simulink model "SimulationForFigure7"  (R2024a)
settings: Solver=ode23tb  StartTime=0.0  StopTime=10.0  RelTol=1e-3
values from neighbouring files (symbols this model uses):
  C_f = 4e-3    (= 0.004)    [necessary_parameter_for_GFM.m]
  C_f_base = 1/(w_nom*Z_base)    (= 0.039788735773)    [necessary_parameter_for_GFM.m]
  kpw = (0.5*2*pi)/1e6    (= 3.14159265359e-06)    [necessary_parameter_for_GFM.m]
  kqv = 20/(1e6)    (= 2e-05)    [necessary_parameter_for_GFM.m]
  L_f = 8e-6    (= 8e-06)    [necessary_parameter_for_GFM.m]
  L_f_base = Z_base/w_nom    (= 0.000254647908947)    [necessary_parameter_for_GFM.m]
  L_g = Length*L_g_per_km    (= 0.005)    [necessary_parameter_for_GFM.m]
  R_f = 1e-4    (= 0.0001)    [necessary_parameter_for_GFM.m]
  R_g = Length*R_g_per_km    (= 0.75)    [necessary_parameter_for_GFM.m]
  V_dc = 1000    [necessary_parameter_for_GFM.m]
  w_nom = 2*pi*f_nom    (= 314.159265359)    [necessary_parameter_for_GFM.m]
libraries: spsabctodq0Lib x8, slpidlib x8, dspstat3 x8, spsThreePhaseSeriesRLCLoadLib x8, spsVoltageMeasurementLib x8, spsThreePhaseSeriesRLCBranchLib x6, spsThreePhaseBreakerLib x6, spsPower3phInstantaneousLib x4, spsThreePhaseVIMeasurementLib x4, cstblocks x4, spsDCVoltageSourceLib x2, spsdq0toabcLib x2
(part 1 of 2)
settings Model: Creator=USER  LastModifiedBy=USER
settings DebuggingCC: AlgebraicLoopMsg=none

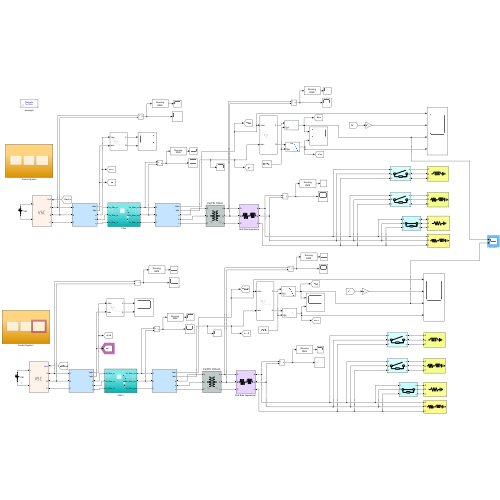
[thumbnail: Simulink's stored preview of the top-level diagram]
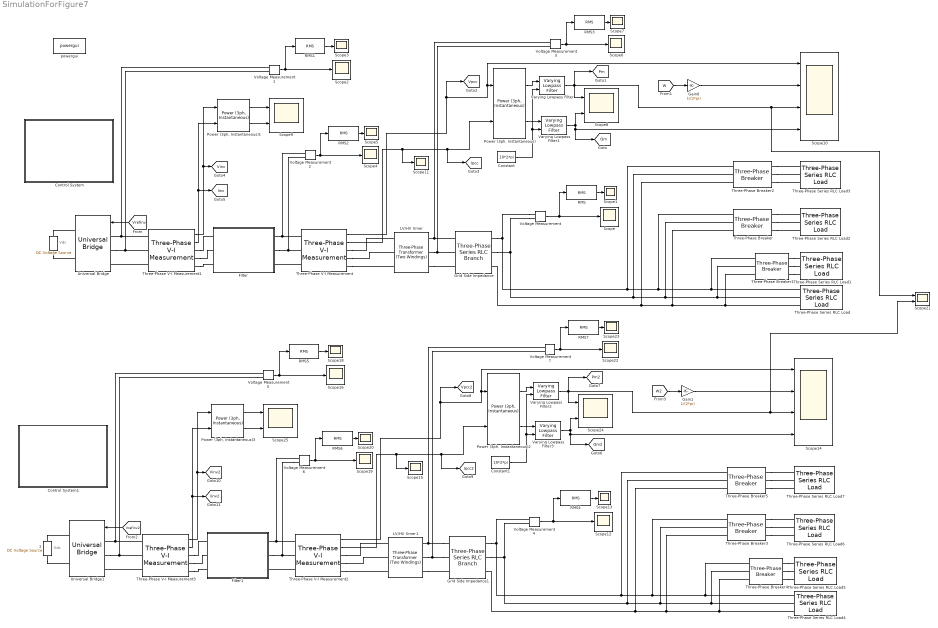
== system SimulationForFigure7 ==
  note: Vdc
  note: Vdc
  "               " : spsDCVoltageSourceLib/DC Voltage Source  Amplitude=V_dc  Measurements=None
  "               1" : spsDCVoltageSourceLib/DC Voltage Source  Amplitude=V_dc  Measurements=None
  Constant : Constant  Value=10*2*pi
  Constant1 : Constant  Value=10*2*pi
  Control System : Subsystem
  Control System1 : Subsystem
  Filter : Subsystem
  Filter1 : Subsystem
  Gain1 : Gain  Gain=1/(2*pi)
  Gain6 : Gain  Gain=1/(2*pi)
  Grid Side Impedance : spsThreePhaseSeriesRLCBranchLib/Three-Phase Series RLC Branch  LConnTagsString=A|B|C  RConnTagsString=A|B|C  BranchType=RL  Resistance=R_g  Inductance=L_g  Capacitance=1e-6  Measurements=None
  Grid Side Impedance1 : spsThreePhaseSeriesRLCBranchLib/Three-Phase Series RLC Branch  LConnTagsString=A|B|C  RConnTagsString=A|B|C  BranchType=RL  Resistance=R_g  Inductance=L_g  Capacitance=1e-6  Measurements=None
  LV/HV Xmer : spsThreePhaseTransformerTwoWindingsLib/Three-Phase Transformer (Two Windings)  Winding1Connection=Yg  Winding2Connection=Yg  CoreType=Three single-phase transformers  SetSaturation=off  Hysteresis=off  DataFile='hysteresis'  SetInitialFlux=off  Measurements=None  UNITS=SI  NominalPower=[ 2000000 50 ]  Winding1=[400 0 0]  Winding2=[33000 0 0]  Rm=inf  Lm=inf  L0=0.5  Saturation=[0 0;20.412 1.2475;4082.5 1.4554]  InitialFluxes=[ 0.8 , -0.8 , 0.7 ]  BreakLoop=off  DiscreteSolver=Trapezoidal iterative  DataType=on  TransfoNumber=0
  LV/HV Xmer1 : spsThreePhaseTransformerTwoWindingsLib/Three-Phase Transformer (Two Windings)  Winding1Connection=Yg  Winding2Connection=Yg  CoreType=Three single-phase transformers  SetSaturation=off  Hysteresis=off  DataFile='hysteresis'  SetInitialFlux=off  Measurements=None  UNITS=SI  NominalPower=[ 2000000 50 ]  Winding1=[400 0 0]  Winding2=[33000 0 0]  Rm=inf  Lm=inf  L0=0.5  Saturation=[0 0;20.412 1.2475;4082.5 1.4554]  InitialFluxes=[ 0.8 , -0.8 , 0.7 ]  BreakLoop=off  DiscreteSolver=Trapezoidal iterative  DataType=on  TransfoNumber=0
  Power (3ph, Instantaneous){,1..3} (4 alike) : spsPower3phInstantaneousLib/Power (3ph, Instantaneous)
  RMS{,1..7} (8 alike) : dspstat3/RMS  run=on  directionMode=Each column  dimension=1  InputProcessing=Columns as channels (frame based)  reset_popup=None
  Scope{,1..7,11..13,15..16,18..20,22..23} (18 alike) : Scope
  Scope10 : Scope  NumInputPorts=4
  Scope14 : Scope  NumInputPorts=4
  Scope{8..9,21,24..25} (5 alike) : Scope  NumInputPorts=2
  Three-Phase Series RLC Load : spsThreePhaseSeriesRLCLoadLib/Three-Phase Series RLC Load  LConnTagsString=A|B|C  Configuration=Y (grounded)  NominalVoltage=33000  Vabc=[1e3 1e3 1e3]  Vabcp=[1e3 1e3 1e3]  NominalFrequency=50  UnbalancedPower=off  ActivePower=0.9e6  InductivePower=4e5  CapacitivePower=0  Pabc=[10e3 9e3 11e3]  QLabc=[100 90 110]  QCabc=[100 90 110]  Pabcp=[10e3 9e3 11e3]  QLabcp=[100 90 110]  QCabcp=[100 90 110]  Measurements=None  LoadType=constant Z
  Three-Phase Series RLC Load1 : spsThreePhaseSeriesRLCLoadLib/Three-Phase Series RLC Load  LConnTagsString=A|B|C  Configuration=Y (grounded)  NominalVoltage=33000  Vabc=[1e3 1e3 1e3]  Vabcp=[1e3 1e3 1e3]  NominalFrequency=50  UnbalancedPower=off  ActivePower=0.1e6  InductivePower=0  CapacitivePower=0  Pabc=[10e3 9e3 11e3]  QLabc=[100 90 110]  QCabc=[100 90 110]  Pabcp=[10e3 9e3 11e3]  QLabcp=[100 90 110]  QCabcp=[100 90 110]  Measurements=None  LoadType=constant Z
  Three-Phase Series RLC Load2 : spsThreePhaseSeriesRLCLoadLib/Three-Phase Series RLC Load  LConnTagsString=A|B|C  Configuration=Y (grounded)  NominalVoltage=33000  Vabc=[1e3 1e3 1e3]  Vabcp=[1e3 1e3 1e3]  NominalFrequency=50  UnbalancedPower=off  ActivePower=0.2e6  InductivePower=4e5  CapacitivePower=0  Pabc=[10e3 9e3 11e3]  QLabc=[100 90 110]  QCabc=[100 90 110]  Pabcp=[10e3 9e3 11e3]  QLabcp=[100 90 110]  QCabcp=[100 90 110]  Measurements=None  LoadType=constant Z
  Three-Phase Series RLC Load3 : spsThreePhaseSeriesRLCLoadLib/Three-Phase Series RLC Load  LConnTagsString=A|B|C  Configuration=Y (grounded)  NominalVoltage=33000  Vabc=[1e3 1e3 1e3]  Vabcp=[1e3 1e3 1e3]  NominalFrequency=50  UnbalancedPower=off  ActivePower=0  InductivePower=1e5  CapacitivePower=0  Pabc=[10e3 9e3 11e3]  QLabc=[100 90 110]  QCabc=[100 90 110]  Pabcp=[10e3 9e3 11e3]  QLabcp=[100 90 110]  QCabcp=[100 90 110]  Measurements=None  LoadType=constant Z
  Three-Phase Series RLC Load4 : spsThreePhaseSeriesRLCLoadLib/Three-Phase Series RLC Load  LConnTagsString=A|B|C  Configuration=Y (grounded)  NominalVoltage=33000  Vabc=[1e3 1e3 1e3]  Vabcp=[1e3 1e3 1e3]  NominalFrequency=50  UnbalancedPower=off  ActivePower=0.9e6  InductivePower=4e5  CapacitivePower=0  Pabc=[10e3 9e3 11e3]  QLabc=[100 90 110]  QCabc=[100 90 110]  Pabcp=[10e3 9e3 11e3]  QLabcp=[100 90 110]  QCabcp=[100 90 110]  Measurements=None  LoadType=constant Z
  Three-Phase Series RLC Load5 : spsThreePhaseSeriesRLCLoadLib/Three-Phase Series RLC Load  LConnTagsString=A|B|C  Configuration=Y (grounded)  NominalVoltage=33000  Vabc=[1e3 1e3 1e3]  Vabcp=[1e3 1e3 1e3]  NominalFrequency=50  UnbalancedPower=off  ActivePower=0.1e6  InductivePower=0  CapacitivePower=0  Pabc=[10e3 9e3 11e3]  QLabc=[100 90 110]  QCabc=[100 90 110]  Pabcp=[10e3 9e3 11e3]  QLabcp=[100 90 110]  QCabcp=[100 90 110]  Measurements=None  LoadType=constant Z
  Three-Phase Series RLC Load6 : spsThreePhaseSeriesRLCLoadLib/Three-Phase Series RLC Load  LConnTagsString=A|B|C  Configuration=Y (grounded)  NominalVoltage=33000  Vabc=[1e3 1e3 1e3]  Vabcp=[1e3 1e3 1e3]  NominalFrequency=50  UnbalancedPower=off  ActivePower=0.2e6  InductivePower=4e5  CapacitivePower=0  Pabc=[10e3 9e3 11e3]  QLabc=[100 90 110]  QCabc=[100 90 110]  Pabcp=[10e3 9e3 11e3]  QLabcp=[100 90 110]  QCabcp=[100 90 110]  Measurements=None  LoadType=constant Z
  Three-Phase Series RLC Load7 : spsThreePhaseSeriesRLCLoadLib/Three-Phase Series RLC Load  LConnTagsString=A|B|C  Configuration=Y (grounded)  NominalVoltage=33000  Vabc=[1e3 1e3 1e3]  Vabcp=[1e3 1e3 1e3]  NominalFrequency=50  UnbalancedPower=off  ActivePower=0  InductivePower=1e5  CapacitivePower=0  Pabc=[10e3 9e3 11e3]  QLabc=[100 90 110]  QCabc=[100 90 110]  Pabcp=[10e3 9e3 11e3]  QLabcp=[100 90 110]  QCabcp=[100 90 110]  Measurements=None  LoadType=constant Z
  Three-Phase V-I Measurement{,1..3} (4 alike) : spsThreePhaseVIMeasurementLib/Three-Phase V-I Measurement  VoltageMeasurement=phase-to-ground  SetLabelV=off  LabelV=Vabc  Vpu=off  VpuLL=off  CurrentMeasurement=yes  SetLabelI=off  LabelI=Iabc  Ipu=off  Pbase=100e6  Vbase=500e3  OutputType=Complex  PhasorSimulation=off  PSBequivalent=0
  Three-Phase Breaker : spsThreePhaseBreakerLib/Three-Phase Breaker  InitialState=open  SwitchA=on  SwitchB=on  SwitchC=on  SwitchTimes="[2  3]"  External=off  BreakerResistance=0.001  SnubberResistance=1e6  SnubberCapacitance=inf  Measurements=None
  Three-Phase Breaker1 : spsThreePhaseBreakerLib/Three-Phase Breaker  InitialState=closed  SwitchA=on  SwitchB=on  SwitchC=on  SwitchTimes=[6 8]  External=off  BreakerResistance=0.001  SnubberResistance=1e6  SnubberCapacitance=inf  Measurements=None
  Three-Phase Breaker2 : spsThreePhaseBreakerLib/Three-Phase Breaker  InitialState=open  SwitchA=on  SwitchB=on  SwitchC=on  SwitchTimes="[4  5]"  External=off  BreakerResistance=0.001  SnubberResistance=1e6  SnubberCapacitance=inf  Measurements=None
  Three-Phase Breaker3 : spsThreePhaseBreakerLib/Three-Phase Breaker  InitialState=open  SwitchA=on  SwitchB=on  SwitchC=on  SwitchTimes="[2  3]"  External=off  BreakerResistance=0.001  SnubberResistance=1e6  SnubberCapacitance=inf  Measurements=None
  Three-Phase Breaker4 : spsThreePhaseBreakerLib/Three-Phase Breaker  InitialState=closed  SwitchA=on  SwitchB=on  SwitchC=on  SwitchTimes=[6 8]  External=off  BreakerResistance=0.001  SnubberResistance=1e6  SnubberCapacitance=inf  Measurements=None
  Three-Phase Breaker5 : spsThreePhaseBreakerLib/Three-Phase Breaker  InitialState=open  SwitchA=on  SwitchB=on  SwitchC=on  SwitchTimes="[4  5]"  External=off  BreakerResistance=0.001  SnubberResistance=1e6  SnubberCapacitance=inf  Measurements=None
  Universal Bridge : spsUniversalBridgeLib/Universal Bridge  Arms=3  SnubberResistance=1e5  SnubberCapacitance=inf  Device=Average-model based VSC  Ron=1e-3  Lon=0  ForwardVoltages="[  0  0  ]"  ForwardVoltage=0  GTOparameters=[ 10e-6 , 20e-6 ]  IGBTparameters=[ 1e-6 , 2e-6 ]  Measurements=None  Measurements_2=None  converterType=Rectifier
  Universal Bridge1 : spsUniversalBridgeLib/Universal Bridge  Arms=3  SnubberResistance=1e5  SnubberCapacitance=inf  Device=Average-model based VSC  Ron=1e-3  Lon=0  ForwardVoltages="[  0  0  ]"  ForwardVoltage=0  GTOparameters=[ 10e-6 , 20e-6 ]  IGBTparameters=[ 1e-6 , 2e-6 ]  Measurements=None  Measurements_2=None  converterType=Rectifier
  Varying Lowpass Filter{,1..3} (4 alike) : cstblocks/Linear Parameter Varying/Varying Lowpass Filter  N=2
  Voltage Measurement{,1..7} (8 alike) : spsVoltageMeasurementLib/Voltage Measurement  PhasorSimulation=off  OutputType=Complex  PSBequivalent=0
  powergui : sps_lib/powergui  Priority=1  SimulationMode=Discrete  SampleTime=1e-5  frequency=60  Iterations=50  frequencyindice=0  Pbase=100e6  ErrMax=1e-4  UnitsV=kV  UnitsW=MW  buscounter=0  FunctionMessages=off  echomessages=off  EnableUseOfTLC=off  CurrentSourceSwitches=off  DisableSnubberDevices=off  DisableRonSwitches=off  DisableVfSwitches=off  DisplayEquations=off  AutomaticDiscreteSolvers=off  SolverType=Tustin/Backward Euler (TBE)  Interpol=off  ExternalGateDelay=off  methode=off  Ts=100  x0status=blocks  SPID=on  SwTol=0  HookPort=off  NonlinearTolerance=1e-4  nMaxIteration=100  ContinueOnMaxIteration=off  RestoreLinks=warning  ResistiveCurrentMeasurement=off  Frange=[0:2:500]  Ylog=off  Xlog=on  ShowGrid=off  save=off  variable=ZData  structure=0  ZoomFFT=off  StartTime=0.0  cycles=1  DisplayStyle=1  fundamental=60  FreqAxis=off  MaxFrequency=1000  frequencyindicesteady=1  RmsSteady=1  display=off
  tag scope: Iinv2=global, Iinv=global, Ipcc2=global, Ipcc=global, Pm2=global, Pm=global, Qm2=global, Qm=global, Vinv2=global, Vinv=global, Vpcc2=global, Vpcc=global
  wires:
  Voltage Measurement1/1 -> RMS1/1, Scope2/1
  RMS/1 -> Scope1/1
  Voltage Measurement/1 -> RMS/1, Scope/1
  RMS2/1 -> Scope5/1
  [Vrefinv] -> Universal Bridge/1
  RMS1/1 -> Scope3/1
  RMS3/1 -> Scope7/1
  Voltage Measurement3/1 -> RMS3/1, Scope6/1
  Voltage Measurement2/1 -> RMS2/1, Scope4/1
  [W] -> Gain6/1
  Three-Phase V-I Measurement/1 -> [Vpcc], Scope10/1, "Power (3ph, Instantaneous)"/1
  Three-Phase V-I Measurement/2 -> Scope11/1, [Ipcc], "Power (3ph, Instantaneous)"/2
  Three-Phase V-I Measurement1/1 -> "Power (3ph, Instantaneous)1"/1, [Vinv]
  Three-Phase V-I Measurement1/2 -> "Power (3ph, Instantaneous)1"/2, [Iinv]
  "Power (3ph, Instantaneous)1"/1 -> Scope9/1
  "Power (3ph, Instantaneous)1"/2 -> Scope9/2
  Gain6/1 -> Scope10/2
  "Power (3ph, Instantaneous)"/2 -> Varying Lowpass Filter1/1
  Varying Lowpass Filter1/1 -> Scope10/4, [Qm], Scope8/2
  Varying Lowpass Filter/1 -> Scope10/3, Scope21/1, Scope8/1, [Pm]
  "Power (3ph, Instantaneous)"/1 -> Varying Lowpass Filter/1
  Constant/1 -> Varying Lowpass Filter1/2, Varying Lowpass Filter/2
  "Power (3ph, Instantaneous)2"/1 -> Varying Lowpass Filter2/1
  Varying Lowpass Filter2/1 -> Scope21/2, Scope14/3, Scope24/1, [Pm2]
  Three-Phase V-I Measurement3/2 -> "Power (3ph, Instantaneous)3"/2, [Iinv2]
  Three-Phase V-I Measurement2/2 -> Scope15/1, [Ipcc2], "Power (3ph, Instantaneous)2"/2
  Three-Phase V-I Measurement2/1 -> [Vpcc2], Scope14/1, "Power (3ph, Instantaneous)2"/1
  RMS4/1 -> Scope13/1
  RMS7/1 -> Scope23/1
  Voltage Measurement4/1 -> RMS4/1, Scope12/1
  Voltage Measurement5/1 -> RMS5/1, Scope16/1
  RMS6/1 -> Scope20/1
  RMS5/1 -> Scope18/1
  Gain1/1 -> Scope14/2
  Constant1/1 -> Varying Lowpass Filter3/2, Varying Lowpass Filter2/2
  Voltage Measurement6/1 -> RMS6/1, Scope19/1
  Varying Lowpass Filter3/1 -> Scope14/4, [Qm2], Scope24/2
  [W2] -> Gain1/1
  Three-Phase V-I Measurement3/1 -> "Power (3ph, Instantaneous)3"/1, [Vinv2]
  Voltage Measurement7/1 -> RMS7/1, Scope22/1
  "Power (3ph, Instantaneous)3"/2 -> Scope25/2
  "Power (3ph, Instantaneous)2"/2 -> Varying Lowpass Filter3/1
  "Power (3ph, Instantaneous)3"/1 -> Scope25/1
  [Vrefinv2] -> Universal Bridge1/1
  connections:
  Voltage Measurement/LConn2 -- Three-Phase Breaker2/LConn2 -- Three-Phase Breaker/LConn2 -- Three-Phase Series RLC Load/LConn2 -- Three-Phase Breaker1/LConn2 -- Grid Side Impedance/RConn2
  Voltage Measurement1/LConn1 -- Universal Bridge/LConn1 -- Three-Phase V-I Measurement1/LConn1
  Universal Bridge/LConn2 -- Three-Phase V-I Measurement1/LConn2 -- Voltage Measurement1/LConn2
  Voltage Measurement/LConn1 -- Three-Phase Breaker2/LConn1 -- Three-Phase Series RLC Load/LConn1 -- Three-Phase Breaker1/LConn1 -- Three-Phase Breaker/LConn1 -- Grid Side Impedance/RConn1
  Filter/RConn2 -- Three-Phase V-I Measurement/LConn2 -- Voltage Measurement2/LConn2
  Voltage Measurement2/LConn1 -- Three-Phase V-I Measurement/LConn1 -- Filter/RConn1
  "               "/LConn1 -- Universal Bridge/RConn2
  Three-Phase V-I Measurement/LConn3 -- Filter/RConn3
  "               "/RConn1 -- Universal Bridge/RConn1
  Three-Phase V-I Measurement/RConn1 -- LV/HV Xmer/LConn1
  Three-Phase V-I Measurement/RConn2 -- LV/HV Xmer/LConn2
  Three-Phase V-I Measurement/RConn3 -- LV/HV Xmer/LConn3
  LV/HV Xmer/RConn1 -- Voltage Measurement3/LConn1 -- Grid Side Impedance/LConn1
  LV/HV Xmer/RConn2 -- Voltage Measurement3/LConn2 -- Grid Side Impedance/LConn2
  LV/HV Xmer/RConn3 -- Grid Side Impedance/LConn3
  Three-Phase V-I Measurement1/LConn3 -- Universal Bridge/LConn3
  Three-Phase V-I Measurement1/RConn1 -- Filter/LConn1
  Three-Phase V-I Measurement1/RConn2 -- Filter/LConn2
  Three-Phase V-I Measurement1/RConn3 -- Filter/LConn3
  Three-Phase Breaker/LConn3 -- Three-Phase Series RLC Load/LConn3 -- Three-Phase Breaker1/LConn3 -- Three-Phase Breaker2/LConn3 -- Grid Side Impedance/RConn3
  Three-Phase Breaker/RConn3 -- Three-Phase Series RLC Load2/LConn3
  Three-Phase Breaker1/RConn1 -- Three-Phase Series RLC Load1/LConn1
  Three-Phase Breaker1/RConn2 -- Three-Phase Series RLC Load1/LConn2
  Three-Phase Breaker/RConn2 -- Three-Phase Series RLC Load2/LConn2
  Three-Phase Breaker1/RConn3 -- Three-Phase Series RLC Load1/LConn3
  Three-Phase Breaker/RConn1 -- Three-Phase Series RLC Load2/LConn1
  Three-Phase Breaker2/RConn1 -- Three-Phase Series RLC Load3/LConn1
  Three-Phase Breaker2/RConn2 -- Three-Phase Series RLC Load3/LConn2
  Three-Phase Breaker2/RConn3 -- Three-Phase Series RLC Load3/LConn3
  Filter1/RConn1 -- Voltage Measurement6/LConn1 -- Three-Phase V-I Measurement2/LConn1
  Three-Phase Breaker3/LConn1 -- Voltage Measurement4/LConn1 -- Grid Side Impedance1/RConn1 -- Three-Phase Breaker5/LConn1 -- Three-Phase Series RLC Load4/LConn1 -- Three-Phase Breaker4/LConn1
  Voltage Measurement5/LConn2 -- Universal Bridge1/LConn2 -- Three-Phase V-I Measurement3/LConn2
  Grid Side Impedance1/RConn2 -- Voltage Measurement4/LConn2 -- Three-Phase Breaker5/LConn2 -- Three-Phase Breaker3/LConn2 -- Three-Phase Series RLC Load4/LConn2 -- Three-Phase Breaker4/LConn2
  Grid Side Impedance1/LConn2 -- LV/HV Xmer1/RConn2 -- Voltage Measurement7/LConn2
  Grid Side Impedance1/LConn1 -- LV/HV Xmer1/RConn1 -- Voltage Measurement7/LConn1
  Three-Phase V-I Measurement3/LConn1 -- Voltage Measurement5/LConn1 -- Universal Bridge1/LConn1
  Three-Phase Breaker4/LConn3 -- Three-Phase Series RLC Load4/LConn3 -- Three-Phase Breaker5/LConn3 -- Grid Side Impedance1/RConn3 -- Three-Phase Breaker3/LConn3
  Voltage Measurement6/LConn2 -- Filter1/RConn2 -- Three-Phase V-I Measurement2/LConn2
  Three-Phase V-I Measurement3/RConn1 -- Filter1/LConn1
  Three-Phase V-I Measurement3/RConn3 -- Filter1/LConn3
  Three-Phase Breaker5/RConn3 -- Three-Phase Series RLC Load7/LConn3
  "               1"/LConn1 -- Universal Bridge1/RConn2
  "               1"/RConn1 -- Universal Bridge1/RConn1
  Three-Phase V-I Measurement2/RConn1 -- LV/HV Xmer1/LConn1
  LV/HV Xmer1/RConn3 -- Grid Side Impedance1/LConn3
  Three-Phase Breaker3/RConn2 -- Three-Phase Series RLC Load6/LConn2
  Three-Phase Breaker5/RConn1 -- Three-Phase Series RLC Load7/LConn1
  Three-Phase Breaker4/RConn3 -- Three-Phase Series RLC Load5/LConn3
  Three-Phase V-I Measurement3/LConn3 -- Universal Bridge1/LConn3
  Three-Phase Breaker4/RConn1 -- Three-Phase Series RLC Load5/LConn1
  Three-Phase Breaker5/RConn2 -- Three-Phase Series RLC Load7/LConn2
  Three-Phase Breaker4/RConn2 -- Three-Phase Series RLC Load5/LConn2
  Three-Phase V-I Measurement2/LConn3 -- Filter1/RConn3
  Three-Phase V-I Measurement3/RConn2 -- Filter1/LConn2
  Three-Phase V-I Measurement2/RConn2 -- LV/HV Xmer1/LConn2
  Three-Phase V-I Measurement2/RConn3 -- LV/HV Xmer1/LConn3
  Three-Phase Breaker3/RConn1 -- Three-Phase Series RLC Load6/LConn1
  Three-Phase Breaker3/RConn3 -- Three-Phase Series RLC Load6/LConn3

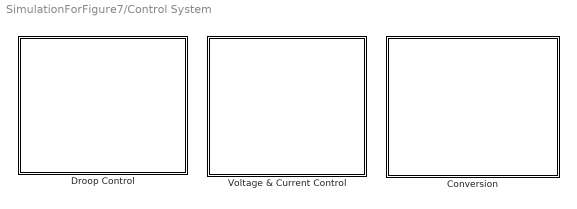
== system SimulationForFigure7/Control System ==
  Conversion : Subsystem
  Droop Control : Subsystem
  Voltage & Current Control : Subsystem

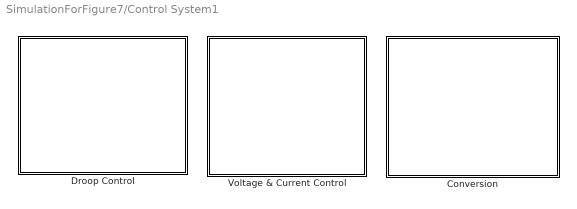
== system SimulationForFigure7/Control System1 ==
  Conversion : Subsystem
  Droop Control : Subsystem
  Voltage & Current Control : Subsystem

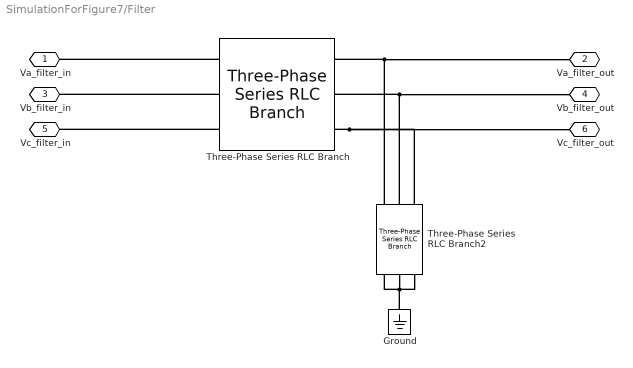
== system SimulationForFigure7/Filter ==
  Ground : spsGroundLib/Ground  LConnTagsString=a
  Three-Phase Series RLC Branch : spsThreePhaseSeriesRLCBranchLib/Three-Phase Series RLC Branch  LConnTagsString=A|B|C  RConnTagsString=A|B|C  BranchType=RL  Resistance=R_f  Inductance=L_f  Capacitance=1e-6  Measurements=None
  Three-Phase Series RLC Branch2 : spsThreePhaseSeriesRLCBranchLib/Three-Phase Series RLC Branch  LConnTagsString=A|B|C  RConnTagsString=A|B|C  BranchType=C  Resistance=1  Inductance=1e-3  Capacitance=C_f  Measurements=None
  Va_filter_in : PMIOPort  Side=Left
  Va_filter_out : PMIOPort  Port=2  Side=Right
  Vb_filter_in : PMIOPort  Port=3  Side=Left
  Vb_filter_out : PMIOPort  Port=4  Side=Right
  Vc_filter_in : PMIOPort  Port=5  Side=Left
  Vc_filter_out : PMIOPort  Port=6  Side=Right
  connections:
  Three-Phase Series RLC Branch2/RConn3 -- Ground/LConn1 -- Three-Phase Series RLC Branch2/RConn2 -- Three-Phase Series RLC Branch2/RConn1
  Three-Phase Series RLC Branch2/LConn2 -- Vb_filter_out/RConn1 -- Three-Phase Series RLC Branch/RConn2
  Three-Phase Series RLC Branch/RConn3 -- Vc_filter_out/RConn1 -- Three-Phase Series RLC Branch2/LConn3
  Three-Phase Series RLC Branch2/LConn1 -- Va_filter_out/RConn1 -- Three-Phase Series RLC Branch/RConn1
  Three-Phase Series RLC Branch/LConn3 -- Vc_filter_in/RConn1
  Three-Phase Series RLC Branch/LConn2 -- Vb_filter_in/RConn1
  Three-Phase Series RLC Branch/LConn1 -- Va_filter_in/RConn1

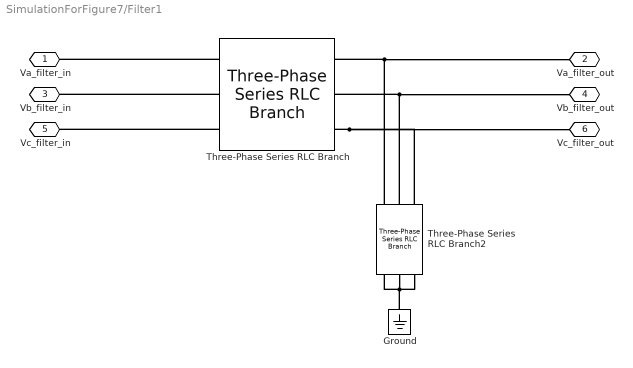
== system SimulationForFigure7/Filter1 ==
  Ground : spsGroundLib/Ground  LConnTagsString=a
  Three-Phase Series RLC Branch : spsThreePhaseSeriesRLCBranchLib/Three-Phase Series RLC Branch  LConnTagsString=A|B|C  RConnTagsString=A|B|C  BranchType=RL  Resistance=R_f  Inductance=L_f  Capacitance=1e-6  Measurements=None
  Three-Phase Series RLC Branch2 : spsThreePhaseSeriesRLCBranchLib/Three-Phase Series RLC Branch  LConnTagsString=A|B|C  RConnTagsString=A|B|C  BranchType=C  Resistance=1  Inductance=1e-3  Capacitance=C_f  Measurements=None
  Va_filter_in : PMIOPort  Side=Left
  Va_filter_out : PMIOPort  Port=2  Side=Right
  Vb_filter_in : PMIOPort  Port=3  Side=Left
  Vb_filter_out : PMIOPort  Port=4  Side=Right
  Vc_filter_in : PMIOPort  Port=5  Side=Left
  Vc_filter_out : PMIOPort  Port=6  Side=Right
  connections:
  Three-Phase Series RLC Branch2/RConn3 -- Ground/LConn1 -- Three-Phase Series RLC Branch2/RConn2 -- Three-Phase Series RLC Branch2/RConn1
  Three-Phase Series RLC Branch2/LConn2 -- Vb_filter_out/RConn1 -- Three-Phase Series RLC Branch/RConn2
  Three-Phase Series RLC Branch/RConn3 -- Vc_filter_out/RConn1 -- Three-Phase Series RLC Branch2/LConn3
  Three-Phase Series RLC Branch2/LConn1 -- Va_filter_out/RConn1 -- Three-Phase Series RLC Branch/RConn1
  Three-Phase Series RLC Branch/LConn3 -- Vc_filter_in/RConn1
  Three-Phase Series RLC Branch/LConn2 -- Vb_filter_in/RConn1
  Three-Phase Series RLC Branch/LConn1 -- Va_filter_in/RConn1

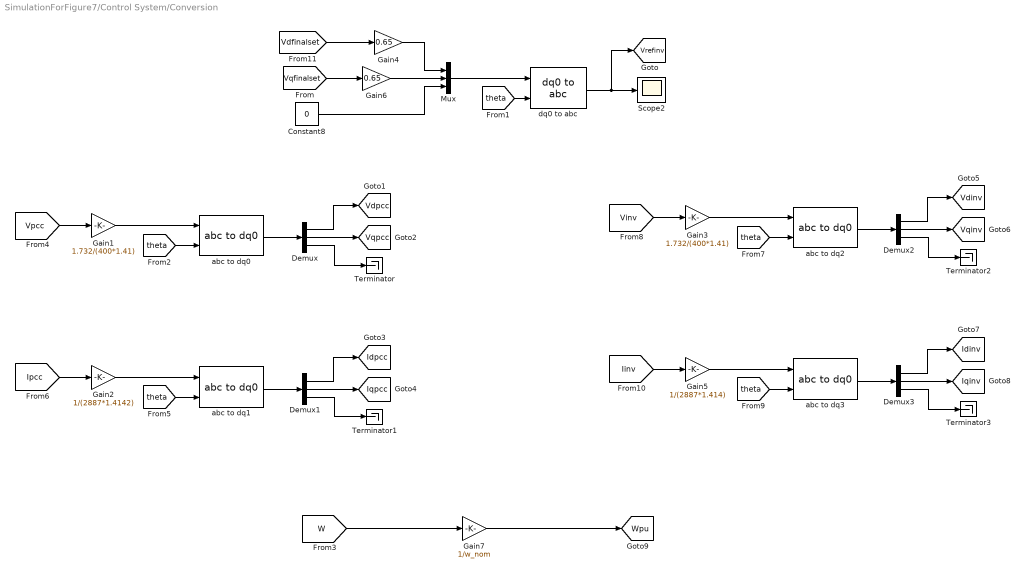
== system SimulationForFigure7/Control System/Conversion ==
  Constant8 : Constant  Value=0
  Demux{,1..3} (4 alike) : Demux  Outputs=3
  Gain1 : Gain  Gain=1.732/(400*1.41)
  Gain2 : Gain  Gain=1/(2887*1.4142)
  Gain3 : Gain  Gain=1.732/(400*1.41)
  Gain4 : Gain  Gain=0.65
  Gain5 : Gain  Gain=1/(2887*1.414)
  Gain6 : Gain  Gain=0.65
  Gain7 : Gain  Gain=1/w_nom
  Mux : Mux  Inputs=3
  Scope2 : Scope
  Terminator{,1..3} (4 alike) : Terminator
  abc to dq{0..3} (4 alike) : spsabctodq0Lib/abc to dq0  Alignment=90 degrees behind phase A axis
  dq0 to abc : spsdq0toabcLib/dq0 to abc  Alignment=90 degrees behind phase A axis
  tag scope: Idinv=global, Idpcc=global, Iqinv=global, Iqpcc=global, Vdinv=global, Vdpcc=global, Vqinv=global, Vqpcc=global, Vrefinv=global, Wpu=global
  wires:
  Constant8/1 -> Mux/3
  Mux/1 -> dq0 to abc/1
  dq0 to abc/1 -> Scope2/1, [Vrefinv]
  Gain4/1 -> Mux/1
  [theta] -> dq0 to abc/2
  [Vqfinalset] -> Gain6/1
  [Vpcc] -> Gain1/1
  [theta] -> abc to dq0/2
  Gain1/1 -> abc to dq0/1
  abc to dq0/1 -> Demux/1
  Demux/1 -> [Vdpcc]
  Demux/2 -> [Vqpcc]
  Demux/3 -> Terminator/1
  [Ipcc] -> Gain2/1
  [theta] -> abc to dq1/2
  Demux1/2 -> [Iqpcc]
  Gain2/1 -> abc to dq1/1
  Demux1/3 -> Terminator1/1
  Demux1/1 -> [Idpcc]
  abc to dq1/1 -> Demux1/1
  abc to dq3/1 -> Demux3/1
  [Iinv] -> Gain5/1
  Demux3/3 -> Terminator3/1
  Demux3/2 -> [Iqinv]
  Demux3/1 -> [Idinv]
  Gain5/1 -> abc to dq3/1
  [Vinv] -> Gain3/1
  [theta] -> abc to dq3/2
  [theta] -> abc to dq2/2
  Gain3/1 -> abc to dq2/1
  Demux2/2 -> [Vqinv]
  Demux2/3 -> Terminator2/1
  Demux2/1 -> [Vdinv]
  abc to dq2/1 -> Demux2/1
  [Vdfinalset] -> Gain4/1
  Gain6/1 -> Mux/2
  [W] -> Gain7/1
  Gain7/1 -> [Wpu]

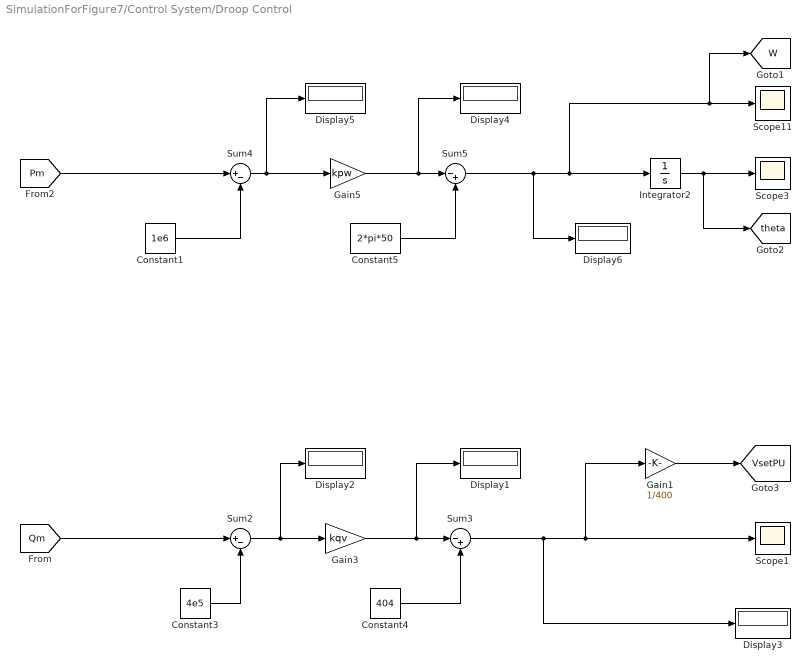
== system SimulationForFigure7/Control System/Droop Control ==
  Constant1 : Constant  Value=1e6
  Constant3 : Constant  Value=4e5
  Constant4 : Constant  Value=404
  Constant5 : Constant  Value=2*pi*50
  Display{1..6} (6 alike) : Display
  Gain1 : Gain  Gain=1/400
  Gain3 : Gain  Gain=kqv
  Gain5 : Gain  Gain=kpw
  Integrator2 : Integrator
  Scope1 : Scope
  Scope11 : Scope
  Scope3 : Scope
  Sum2 : Sum  Inputs=|+-
  Sum3 : Sum  Inputs=|-+
  Sum4 : Sum  Inputs=|+-
  Sum5 : Sum  Inputs=|-+
  tag scope: VsetPU=global, W=global, theta=global
  wires:
  Sum4/1 -> Display5/1, Gain5/1
  Gain5/1 -> Display4/1, Sum5/1
  Gain3/1 -> Sum3/1, Display1/1
  Sum2/1 -> Gain3/1, Display2/1
  Constant5/1 -> Sum5/2
  Constant4/1 -> Sum3/2
  Integrator2/1 -> [theta], Scope3/1
  Constant1/1 -> Sum4/2
  Constant3/1 -> Sum2/2
  Gain1/1 -> [VsetPU]
  [Pm] -> Sum4/1
  [Qm] -> Sum2/1
  Sum5/1 -> Integrator2/1, Scope11/1, [W], Display6/1
  Sum3/1 -> Scope1/1, Gain1/1, Display3/1

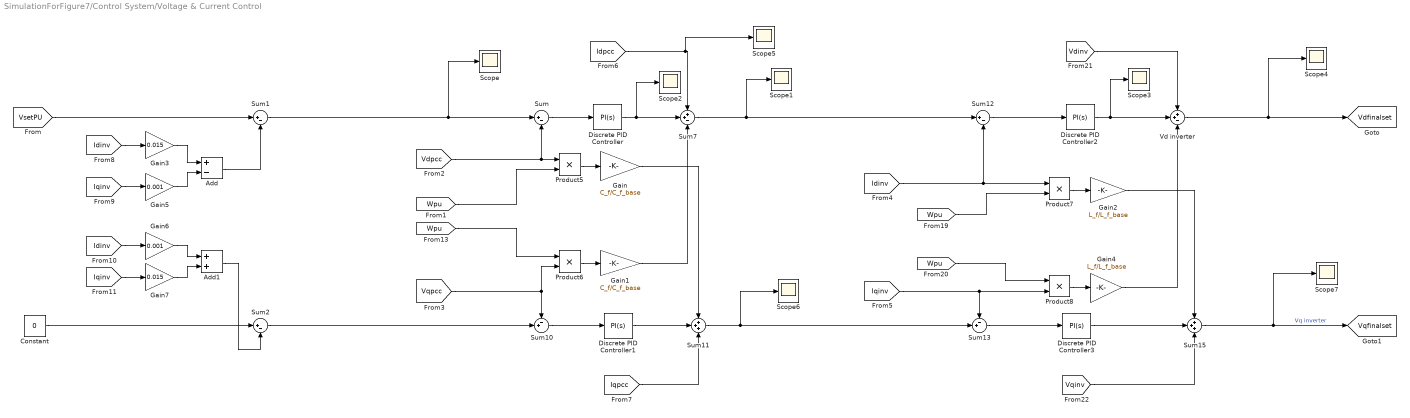
== system SimulationForFigure7/Control System/Voltage & Current Control ==
  Add : Sum  Inputs=+-
  Add1 : Sum
  Constant : Constant  Value=0
  Discrete PID Controller : slpidlib/PID Controller  Controller=PI  Form=Parallel  TimeDomain=Continuous-time  UseExternalTs=off  SampleTime=1e-4  IntegratorMethod=Forward Euler  FilterMethod=Forward Euler  ControllerParametersSource=internal  P=5  I=10  UseKiTs=off  D=0  UseExternalDerivativeSource=off  N=100  UseFilter=on  TunerSelectOption=Transfer Function Based (PID Tuner App)  InitialConditionSource=internal  InitialConditionForIntegrator=0  InitialConditionForFilter=0  DifferentiatorICPrevScaledInput=0  ExternalReset=none  TrackingMode=off  Kt=1  LimitOutput=off  SatLimitsSource=internal  UpperSaturationLimit=inf  LowerSaturationLimit=-inf  LinearizeAsGain=off  AntiWindupMode=none  Kb=1  LimitIntegrator=off  UpperIntegratorSaturationLimit=inf  LowerIntegratorSaturationLimit=-inf  POutMin=[]  POutMax=[]  IOutMin=[]  IOutMax=[]  DOutMin=[]  DOutMax=[]  NOutMin=[]  NOutMax=[]  SumOutMin=[]  SumOutMax=[]  SaturationOutMin=[]  SaturationOutMax=[]  PParamMin=[]  PParamMax=[]  IParamMin=[]  IParamMax=[]  DParamMin=[]  DParamMax=[]  NParamMin=[]  NParamMax=[]  KbParamMin=[]  KbParamMax=[]  KtParamMin=[]  KtParamMax=[]  KbOutMin=[]  KbOutMax=[]  KtOutMin=[]  KtOutMax=[]  IntegratorOutMin=[]  IntegratorOutMax=[]  FilterOutMin=[]  FilterOutMax=[]  SumI1OutMin=[]  SumI1OutMax=[]  SumI2OutMin=[]  SumI2OutMax=[]  SumI3OutMin=[]  SumI3OutMax=[]  SumI4OutMin=[]  SumI4OutMax=[]  SumDOutMin=[]  SumDOutMax=[]  DifferentiatorOutMin=[]  DifferentiatorOutMax=[]  FilterDiffOutCoefMin=[]  FilterDiffOutCoefMax=[]  ReciprocalOutMin=[]  ReciprocalOutMax=[]  SumDenOutMin=[]  SumDenOutMax=[]  SumNumOutMin=[]  SumNumOutMax=[]  DivideOutMin=[]  DivideOutMax=[]  UdiffTsProdOutMin=[]  UdiffTsProdOutMax=[]  NTsProdOutMin=[]  NTsProdOutMax=[]  UintegralTsProdOutMin=[]  UintegralTsProdOutMax=[]  UngainTsProdOutMin=[]  UngainTsProdOutMax=[]  ClampingZeroOutDataTypeStr=Inherit: Inherit via back propagation  ClampingZeroOutMin=[]  ClampingZeroOutMax=[]  FilterDenConstantOutDataTypeStr=Inherit: Inherit via back propagation  FilterDenConstantOutMin=[]  FilterDenConstantOutMax=[]  PCopyOutDataTypeStr=Inherit: Inherit via back propagation  PCopyOutMin=[]  PCopyOutMax=[]  NCopyOutDataTypeStr=Inherit: Inherit via back propagation  NCopyOutMin=[]  NCopyOutMax=[]  IntegratorContinuousStateAttributes=''  IntegratorStateMustResolveToSignalObject=off  IntegratorRTWStateStorageClass=Auto  FilterContinuousStateAttributes=''  FilterStateMustResolveToSignalObject=off  FilterRTWStateStorageClass=Auto  ParallelPVariant=InternalParameters  IdealPVariant=Disabled  IVariant=InternalParameters  DVariant=Disabled  IntegratorVariant=Continuous  SatVariant=Disabled  AWVariant=Passthrough  PCopyVariant=Disabled  TRVariant=Disabled  FdbkBlocksVariant=Forward  IdealPFdbkVariant=Disabled  SatFdbkVariant=Disabled  DerivativeFilterVariant=Disabled  NVariant=Disabled  NCopyVariant=Disabled_SignalSpec  FilterICVariant=Disabled  IntegratorICVariant=InternalICs  ExternalResetVariant=Disabled  TRSumVariant=Passthrough  SumFdbkVariant=Disabled  SumVariant=Sum_PI  TsampFilterVariant=InternalTs  TsampNgainVariant=Passthrough  TsampIntegralVariant=Disabled_SignalSpec  ExternalSaturationOutDataTypeStr=Inherit: Same as second input  DerivativeSourceVariant=Disabled
  Discrete PID Controller1 : slpidlib/PID Controller  Controller=PI  Form=Parallel  TimeDomain=Continuous-time  UseExternalTs=off  SampleTime=1e-4  IntegratorMethod=Forward Euler  FilterMethod=Forward Euler  ControllerParametersSource=internal  P=5  I=10  UseKiTs=off  D=0  UseExternalDerivativeSource=off  N=100  UseFilter=on  TunerSelectOption=Transfer Function Based (PID Tuner App)  InitialConditionSource=internal  InitialConditionForIntegrator=0  InitialConditionForFilter=0  DifferentiatorICPrevScaledInput=0  ExternalReset=none  TrackingMode=off  Kt=1  LimitOutput=off  SatLimitsSource=internal  UpperSaturationLimit=inf  LowerSaturationLimit=-inf  LinearizeAsGain=off  AntiWindupMode=none  Kb=1  LimitIntegrator=off  UpperIntegratorSaturationLimit=inf  LowerIntegratorSaturationLimit=-inf  POutMin=[]  POutMax=[]  IOutMin=[]  IOutMax=[]  DOutMin=[]  DOutMax=[]  NOutMin=[]  NOutMax=[]  SumOutMin=[]  SumOutMax=[]  SaturationOutMin=[]  SaturationOutMax=[]  PParamMin=[]  PParamMax=[]  IParamMin=[]  IParamMax=[]  DParamMin=[]  DParamMax=[]  NParamMin=[]  NParamMax=[]  KbParamMin=[]  KbParamMax=[]  KtParamMin=[]  KtParamMax=[]  KbOutMin=[]  KbOutMax=[]  KtOutMin=[]  KtOutMax=[]  IntegratorOutMin=[]  IntegratorOutMax=[]  FilterOutMin=[]  FilterOutMax=[]  SumI1OutMin=[]  SumI1OutMax=[]  SumI2OutMin=[]  SumI2OutMax=[]  SumI3OutMin=[]  SumI3OutMax=[]  SumI4OutMin=[]  SumI4OutMax=[]  SumDOutMin=[]  SumDOutMax=[]  DifferentiatorOutMin=[]  DifferentiatorOutMax=[]  FilterDiffOutCoefMin=[]  FilterDiffOutCoefMax=[]  ReciprocalOutMin=[]  ReciprocalOutMax=[]  SumDenOutMin=[]  SumDenOutMax=[]  SumNumOutMin=[]  SumNumOutMax=[]  DivideOutMin=[]  DivideOutMax=[]  UdiffTsProdOutMin=[]  UdiffTsProdOutMax=[]  NTsProdOutMin=[]  NTsProdOutMax=[]  UintegralTsProdOutMin=[]  UintegralTsProdOutMax=[]  UngainTsProdOutMin=[]  UngainTsProdOutMax=[]  ClampingZeroOutDataTypeStr=Inherit: Inherit via back propagation  ClampingZeroOutMin=[]  ClampingZeroOutMax=[]  FilterDenConstantOutDataTypeStr=Inherit: Inherit via back propagation  FilterDenConstantOutMin=[]  FilterDenConstantOutMax=[]  PCopyOutDataTypeStr=Inherit: Inherit via back propagation  PCopyOutMin=[]  PCopyOutMax=[]  NCopyOutDataTypeStr=Inherit: Inherit via back propagation  NCopyOutMin=[]  NCopyOutMax=[]  IntegratorContinuousStateAttributes=''  IntegratorStateMustResolveToSignalObject=off  IntegratorRTWStateStorageClass=Auto  FilterContinuousStateAttributes=''  FilterStateMustResolveToSignalObject=off  FilterRTWStateStorageClass=Auto  ParallelPVariant=InternalParameters  IdealPVariant=Disabled  IVariant=InternalParameters  DVariant=Disabled  IntegratorVariant=Continuous  SatVariant=Disabled  AWVariant=Passthrough  PCopyVariant=Disabled  TRVariant=Disabled  FdbkBlocksVariant=Forward  IdealPFdbkVariant=Disabled  SatFdbkVariant=Disabled  DerivativeFilterVariant=Disabled  NVariant=Disabled  NCopyVariant=Disabled_SignalSpec  FilterICVariant=Disabled  IntegratorICVariant=InternalICs  ExternalResetVariant=Disabled  TRSumVariant=Passthrough  SumFdbkVariant=Disabled  SumVariant=Sum_PI  TsampFilterVariant=InternalTs  TsampNgainVariant=Passthrough  TsampIntegralVariant=Disabled_SignalSpec  ExternalSaturationOutDataTypeStr=Inherit: Same as second input  DerivativeSourceVariant=Disabled
  Discrete PID Controller2 : slpidlib/PID Controller  Controller=PI  Form=Parallel  TimeDomain=Continuous-time  UseExternalTs=off  SampleTime=1e-4  IntegratorMethod=Forward Euler  FilterMethod=Forward Euler  ControllerParametersSource=internal  P=0.2  I=1  UseKiTs=off  D=0  UseExternalDerivativeSource=off  N=100  UseFilter=on  TunerSelectOption=Transfer Function Based (PID Tuner App)  InitialConditionSource=internal  InitialConditionForIntegrator=0  InitialConditionForFilter=0  DifferentiatorICPrevScaledInput=0  ExternalReset=none  TrackingMode=off  Kt=1  LimitOutput=off  SatLimitsSource=internal  UpperSaturationLimit=inf  LowerSaturationLimit=-inf  LinearizeAsGain=off  AntiWindupMode=none  Kb=1  LimitIntegrator=off  UpperIntegratorSaturationLimit=inf  LowerIntegratorSaturationLimit=-inf  POutMin=[]  POutMax=[]  IOutMin=[]  IOutMax=[]  DOutMin=[]  DOutMax=[]  NOutMin=[]  NOutMax=[]  SumOutMin=[]  SumOutMax=[]  SaturationOutMin=[]  SaturationOutMax=[]  PParamMin=[]  PParamMax=[]  IParamMin=[]  IParamMax=[]  DParamMin=[]  DParamMax=[]  NParamMin=[]  NParamMax=[]  KbParamMin=[]  KbParamMax=[]  KtParamMin=[]  KtParamMax=[]  KbOutMin=[]  KbOutMax=[]  KtOutMin=[]  KtOutMax=[]  IntegratorOutMin=[]  IntegratorOutMax=[]  FilterOutMin=[]  FilterOutMax=[]  SumI1OutMin=[]  SumI1OutMax=[]  SumI2OutMin=[]  SumI2OutMax=[]  SumI3OutMin=[]  SumI3OutMax=[]  SumI4OutMin=[]  SumI4OutMax=[]  SumDOutMin=[]  SumDOutMax=[]  DifferentiatorOutMin=[]  DifferentiatorOutMax=[]  FilterDiffOutCoefMin=[]  FilterDiffOutCoefMax=[]  ReciprocalOutMin=[]  ReciprocalOutMax=[]  SumDenOutMin=[]  SumDenOutMax=[]  SumNumOutMin=[]  SumNumOutMax=[]  DivideOutMin=[]  DivideOutMax=[]  UdiffTsProdOutMin=[]  UdiffTsProdOutMax=[]  NTsProdOutMin=[]  NTsProdOutMax=[]  UintegralTsProdOutMin=[]  UintegralTsProdOutMax=[]  UngainTsProdOutMin=[]  UngainTsProdOutMax=[]  ClampingZeroOutDataTypeStr=Inherit: Inherit via back propagation  ClampingZeroOutMin=[]  ClampingZeroOutMax=[]  FilterDenConstantOutDataTypeStr=Inherit: Inherit via back propagation  FilterDenConstantOutMin=[]  FilterDenConstantOutMax=[]  PCopyOutDataTypeStr=Inherit: Inherit via back propagation  PCopyOutMin=[]  PCopyOutMax=[]  NCopyOutDataTypeStr=Inherit: Inherit via back propagation  NCopyOutMin=[]  NCopyOutMax=[]  IntegratorContinuousStateAttributes=''  IntegratorStateMustResolveToSignalObject=off  IntegratorRTWStateStorageClass=Auto  FilterContinuousStateAttributes=''  FilterStateMustResolveToSignalObject=off  FilterRTWStateStorageClass=Auto  ParallelPVariant=InternalParameters  IdealPVariant=Disabled  IVariant=InternalParameters  DVariant=Disabled  IntegratorVariant=Continuous  SatVariant=Disabled  AWVariant=Passthrough  PCopyVariant=Disabled  TRVariant=Disabled  FdbkBlocksVariant=Forward  IdealPFdbkVariant=Disabled  SatFdbkVariant=Disabled  DerivativeFilterVariant=Disabled  NVariant=Disabled  NCopyVariant=Disabled_SignalSpec  FilterICVariant=Disabled  IntegratorICVariant=InternalICs  ExternalResetVariant=Disabled  TRSumVariant=Passthrough  SumFdbkVariant=Disabled  SumVariant=Sum_PI  TsampFilterVariant=InternalTs  TsampNgainVariant=Passthrough  TsampIntegralVariant=Disabled_SignalSpec  ExternalSaturationOutDataTypeStr=Inherit: Same as second input  DerivativeSourceVariant=Disabled
  Discrete PID Controller3 : slpidlib/PID Controller  Controller=PI  Form=Parallel  TimeDomain=Continuous-time  UseExternalTs=off  SampleTime=1e-4  IntegratorMethod=Forward Euler  FilterMethod=Forward Euler  ControllerParametersSource=internal  P=0.2  I=1  UseKiTs=off  D=0  UseExternalDerivativeSource=off  N=100  UseFilter=on  TunerSelectOption=Transfer Function Based (PID Tuner App)  InitialConditionSource=internal  InitialConditionForIntegrator=0  InitialConditionForFilter=0  DifferentiatorICPrevScaledInput=0  ExternalReset=none  TrackingMode=off  Kt=1  LimitOutput=off  SatLimitsSource=internal  UpperSaturationLimit=inf  LowerSaturationLimit=-inf  LinearizeAsGain=off  AntiWindupMode=none  Kb=1  LimitIntegrator=off  UpperIntegratorSaturationLimit=inf  LowerIntegratorSaturationLimit=-inf  POutMin=[]  POutMax=[]  IOutMin=[]  IOutMax=[]  DOutMin=[]  DOutMax=[]  NOutMin=[]  NOutMax=[]  SumOutMin=[]  SumOutMax=[]  SaturationOutMin=[]  SaturationOutMax=[]  PParamMin=[]  PParamMax=[]  IParamMin=[]  IParamMax=[]  DParamMin=[]  DParamMax=[]  NParamMin=[]  NParamMax=[]  KbParamMin=[]  KbParamMax=[]  KtParamMin=[]  KtParamMax=[]  KbOutMin=[]  KbOutMax=[]  KtOutMin=[]  KtOutMax=[]  IntegratorOutMin=[]  IntegratorOutMax=[]  FilterOutMin=[]  FilterOutMax=[]  SumI1OutMin=[]  SumI1OutMax=[]  SumI2OutMin=[]  SumI2OutMax=[]  SumI3OutMin=[]  SumI3OutMax=[]  SumI4OutMin=[]  SumI4OutMax=[]  SumDOutMin=[]  SumDOutMax=[]  DifferentiatorOutMin=[]  DifferentiatorOutMax=[]  FilterDiffOutCoefMin=[]  FilterDiffOutCoefMax=[]  ReciprocalOutMin=[]  ReciprocalOutMax=[]  SumDenOutMin=[]  SumDenOutMax=[]  SumNumOutMin=[]  SumNumOutMax=[]  DivideOutMin=[]  DivideOutMax=[]  UdiffTsProdOutMin=[]  UdiffTsProdOutMax=[]  NTsProdOutMin=[]  NTsProdOutMax=[]  UintegralTsProdOutMin=[]  UintegralTsProdOutMax=[]  UngainTsProdOutMin=[]  UngainTsProdOutMax=[]  ClampingZeroOutDataTypeStr=Inherit: Inherit via back propagation  ClampingZeroOutMin=[]  ClampingZeroOutMax=[]  FilterDenConstantOutDataTypeStr=Inherit: Inherit via back propagation  FilterDenConstantOutMin=[]  FilterDenConstantOutMax=[]  PCopyOutDataTypeStr=Inherit: Inherit via back propagation  PCopyOutMin=[]  PCopyOutMax=[]  NCopyOutDataTypeStr=Inherit: Inherit via back propagation  NCopyOutMin=[]  NCopyOutMax=[]  IntegratorContinuousStateAttributes=''  IntegratorStateMustResolveToSignalObject=off  IntegratorRTWStateStorageClass=Auto  FilterContinuousStateAttributes=''  FilterStateMustResolveToSignalObject=off  FilterRTWStateStorageClass=Auto  ParallelPVariant=InternalParameters  IdealPVariant=Disabled  IVariant=InternalParameters  DVariant=Disabled  IntegratorVariant=Continuous  SatVariant=Disabled  AWVariant=Passthrough  PCopyVariant=Disabled  TRVariant=Disabled  FdbkBlocksVariant=Forward  IdealPFdbkVariant=Disabled  SatFdbkVariant=Disabled  DerivativeFilterVariant=Disabled  NVariant=Disabled  NCopyVariant=Disabled_SignalSpec  FilterICVariant=Disabled  IntegratorICVariant=InternalICs  ExternalResetVariant=Disabled  TRSumVariant=Passthrough  SumFdbkVariant=Disabled  SumVariant=Sum_PI  TsampFilterVariant=InternalTs  TsampNgainVariant=Passthrough  TsampIntegralVariant=Disabled_SignalSpec  ExternalSaturationOutDataTypeStr=Inherit: Same as second input  DerivativeSourceVariant=Disabled
  Gain : Gain  Gain=C_f/C_f_base
  Gain1 : Gain  Gain=C_f/C_f_base
  Gain2 : Gain  Gain=L_f/L_f_base
  Gain3 : Gain  Gain=0.015
  Gain4 : Gain  Gain=L_f/L_f_base
  Gain5 : Gain  Gain=0.001
  Gain6 : Gain  Gain=0.001
  Gain7 : Gain  Gain=0.015
  Product{5..8} (4 alike) : Product
  Scope{,1..7} (8 alike) : Scope
  Sum{,1..2,12} (4 alike) : Sum  Inputs=|+-
  Sum10 : Sum  Inputs=-+|
  Sum11 : Sum  Inputs=+++
  Sum13 : Sum  Inputs=-+|
  Sum15 : Sum  Inputs=+++
  Sum7 : Sum  Inputs=++-
  Vd inverter : Sum  Inputs=++-
  tag scope: Vdfinalset=global, Vqfinalset=global
  wires:
  [Vdpcc] -> Sum/2, Product5/1
  [Iqpcc] -> Sum11/3
  Discrete PID Controller3/1 -> Sum15/2
  Sum7/1 -> Scope1/1, Sum12/1
  [Iqinv] -> Sum13/1, Product8/2
  Sum15/1 -> Scope7/1, [Vqfinalset]  "Vq inverter"
  Discrete PID Controller2/1 -> Scope3/1, Vd inverter/2
  [Idinv] -> Sum12/2, Product7/1
  [Vqpcc] -> Product6/2, Sum10/1
  [Wpu] -> Product6/1
  Discrete PID Controller1/1 -> Sum11/2
  Product6/1 -> Gain1/1
  Product8/1 -> Gain4/1
  Sum13/1 -> Discrete PID Controller3/1
  Sum12/1 -> Discrete PID Controller2/1
  [Idpcc] -> Scope5/1, Sum7/1
  Sum/1 -> Discrete PID Controller/1
  [Wpu] -> Product7/2
  [Wpu] -> Product5/2
  Sum10/1 -> Discrete PID Controller1/1
  Product5/1 -> Gain/1
  Discrete PID Controller/1 -> Scope2/1, Sum7/2
  [Wpu] -> Product8/1
  Sum11/1 -> Scope6/1, Sum13/2
  Product7/1 -> Gain2/1
  [Vdinv] -> Vd inverter/1
  [Vqinv] -> Sum15/3
  Vd inverter/1 -> Scope4/1, [Vdfinalset]
  Gain4/1 -> Vd inverter/3
  Gain2/1 -> Sum15/1
  Gain/1 -> Sum11/1
  Gain1/1 -> Sum7/3
  Constant/1 -> Sum2/1
  Sum2/1 -> Sum10/2
  Sum1/1 -> Scope/1, Sum/1
  [VsetPU] -> Sum1/1
  Add/1 -> Sum1/2
  [Idinv] -> Gain3/1
  Gain3/1 -> Add/1
  [Iqinv] -> Gain5/1
  Gain5/1 -> Add/2
  [Idinv] -> Gain6/1
  Gain6/1 -> Add1/1
  [Iqinv] -> Gain7/1
  Gain7/1 -> Add1/2
  Add1/1 -> Sum2/2

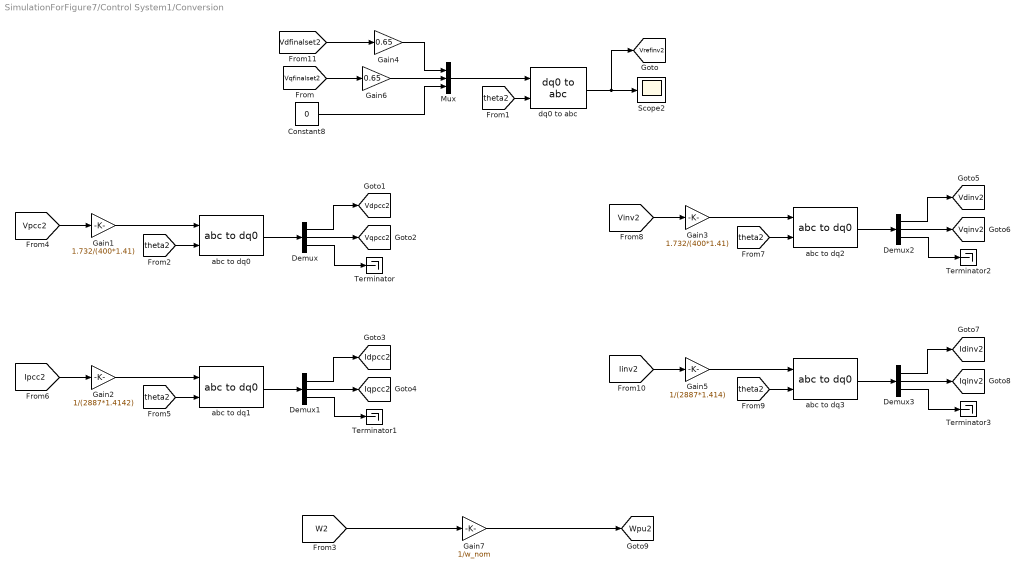
== system SimulationForFigure7/Control System1/Conversion ==
  Constant8 : Constant  Value=0
  Demux{,1..3} (4 alike) : Demux  Outputs=3
  Gain1 : Gain  Gain=1.732/(400*1.41)
  Gain2 : Gain  Gain=1/(2887*1.4142)
  Gain3 : Gain  Gain=1.732/(400*1.41)
  Gain4 : Gain  Gain=0.65
  Gain5 : Gain  Gain=1/(2887*1.414)
  Gain6 : Gain  Gain=0.65
  Gain7 : Gain  Gain=1/w_nom
  Mux : Mux  Inputs=3
  Scope2 : Scope
  Terminator{,1..3} (4 alike) : Terminator
  abc to dq{0..3} (4 alike) : spsabctodq0Lib/abc to dq0  Alignment=90 degrees behind phase A axis
  dq0 to abc : spsdq0toabcLib/dq0 to abc  Alignment=90 degrees behind phase A axis
  tag scope: Idinv2=global, Idpcc2=global, Iqinv2=global, Iqpcc2=global, Vdinv2=global, Vdpcc2=global, Vqinv2=global, Vqpcc2=global, Vrefinv2=global, Wpu2=global
  wires:
  Constant8/1 -> Mux/3
  Mux/1 -> dq0 to abc/1
  dq0 to abc/1 -> Scope2/1, [Vrefinv2]
  Gain4/1 -> Mux/1
  [theta2] -> dq0 to abc/2
  [Vqfinalset2] -> Gain6/1
  [Vpcc2] -> Gain1/1
  [theta2] -> abc to dq0/2
  Gain1/1 -> abc to dq0/1
  abc to dq0/1 -> Demux/1
  Demux/1 -> [Vdpcc2]
  Demux/2 -> [Vqpcc2]
  Demux/3 -> Terminator/1
  [Ipcc2] -> Gain2/1
  [theta2] -> abc to dq1/2
  Demux1/2 -> [Iqpcc2]
  Gain2/1 -> abc to dq1/1
  Demux1/3 -> Terminator1/1
  Demux1/1 -> [Idpcc2]
  abc to dq1/1 -> Demux1/1
  abc to dq3/1 -> Demux3/1
  [Iinv2] -> Gain5/1
  Demux3/3 -> Terminator3/1
  Demux3/2 -> [Iqinv2]
  Demux3/1 -> [Idinv2]
  Gain5/1 -> abc to dq3/1
  [Vinv2] -> Gain3/1
  [theta2] -> abc to dq3/2
  [theta2] -> abc to dq2/2
  Gain3/1 -> abc to dq2/1
  Demux2/2 -> [Vqinv2]
  Demux2/3 -> Terminator2/1
  Demux2/1 -> [Vdinv2]
  abc to dq2/1 -> Demux2/1
  [Vdfinalset2] -> Gain4/1
  Gain6/1 -> Mux/2
  [W2] -> Gain7/1
  Gain7/1 -> [Wpu2]

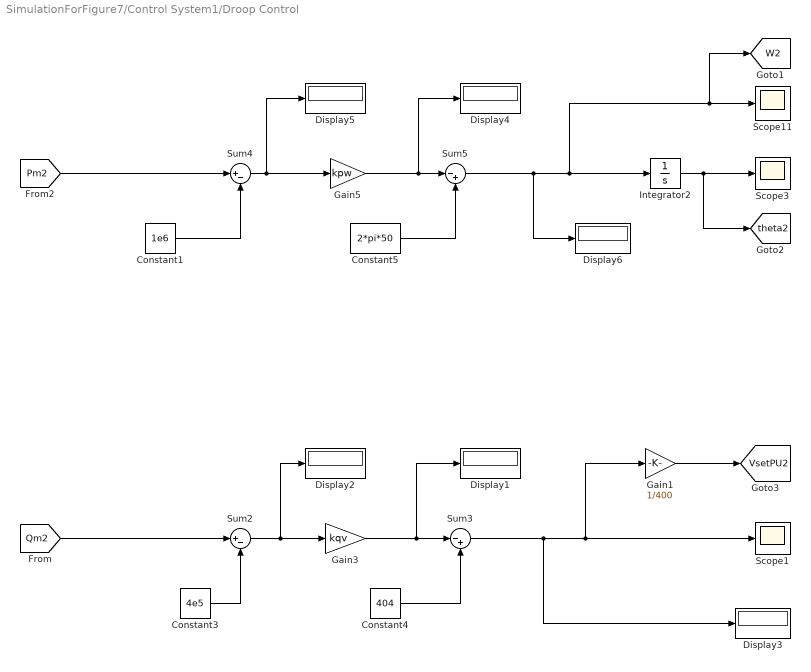
== system SimulationForFigure7/Control System1/Droop Control ==
  Constant1 : Constant  Value=1e6
  Constant3 : Constant  Value=4e5
  Constant4 : Constant  Value=404
  Constant5 : Constant  Value=2*pi*50
  Display{1..6} (6 alike) : Display
  Gain1 : Gain  Gain=1/400
  Gain3 : Gain  Gain=kqv
  Gain5 : Gain  Gain=kpw
  Integrator2 : Integrator
  Scope1 : Scope
  Scope11 : Scope
  Scope3 : Scope
  Sum2 : Sum  Inputs=|+-
  Sum3 : Sum  Inputs=|-+
  Sum4 : Sum  Inputs=|+-
  Sum5 : Sum  Inputs=|-+
  tag scope: VsetPU2=global, W2=global, theta2=global
  wires:
  Sum4/1 -> Display5/1, Gain5/1
  Gain5/1 -> Display4/1, Sum5/1
  Gain3/1 -> Sum3/1, Display1/1
  Sum2/1 -> Gain3/1, Display2/1
  Constant5/1 -> Sum5/2
  Constant4/1 -> Sum3/2
  Integrator2/1 -> [theta2], Scope3/1
  Constant1/1 -> Sum4/2
  Constant3/1 -> Sum2/2
  Gain1/1 -> [VsetPU2]
  [Pm2] -> Sum4/1
  [Qm2] -> Sum2/1
  Sum5/1 -> Integrator2/1, Scope11/1, [W2], Display6/1
  Sum3/1 -> Scope1/1, Gain1/1, Display3/1
